simulink model "Project_model"  (R2024a)
settings: Solver=VariableStepAuto  StartTime=0.0  StopTime=Ts  RelTol=1e-4
values from neighbouring files (symbols this model uses):
  a = L/2    (= 1.385)    [IdeaI_vs_real_braking.m]    (also in Initialization_script.m)
  acc_pedal = 0    [Initialization_script.m]
  Af = 2.36    [Initialization_script.m]
  alpha = 0    [Initialization_script.m]
  b = L-a    (= 1.385)    [IdeaI_vs_real_braking.m]    (also in Initialization_script.m)
  brake_pedal = 1    [Initialization_script.m]
  Cx = 0.27    [Initialization_script.m]
  delay_acc = 0.02    [Initialization_script.m]
  delay_brake = 0.02    [Initialization_script.m]
  delay_release_acc = 30    [Initialization_script.m]
  delay_release_brake = 100    [Initialization_script.m]
  E_max = 58e3    (= 58000)    [Initialization_script.m]    (also in Power_losses.m)
  eff_engine = 0.90    (= 0.9)    [Caratteristica_coppia_rpm.m]    (also in Initialization_script.m)
  eff_transmission = 0.95    [Initialization_script.m]
  f0 = 0.009    [Initialization_script.m]
  f2 = 6.5e-6    (= 6.5e-06)    [Initialization_script.m]
  g = 9.81    [IdeaI_vs_real_braking.m]    (also in Initialization_script.m)
  gamma = 0    [Initialization_script.m]
  gear_ratio = 10.5    [Initialization_script.m]
  h = 0.55    [IdeaI_vs_real_braking.m]    (also in Initialization_script.m)
  Jns = 1    [Initialization_script.m]
  L = 2.77    [IdeaI_vs_real_braking.m]    (also in Initialization_script.m)
  lon_r = 0.055    [Initialization_script.m]    (also in Tyre215_50_19_Comb.m)
  m = 1812    [IdeaI_vs_real_braking.m]    (also in Initialization_script.m)
  max_braking_force = 15*m    (= 27180)    [Initialization_script.m]
  mu = 0.01:0.01:2    [IdeaI_vs_real_braking.m]    (also in Initialization_script.m = mmu(i))
  Pacn = Pace'    [Initialization_script.m]
  Radius = 0.35    [Initialization_script.m]    (also in Power_losses.m)
  regen_scaling = 1/10    (= 0.1)    [Initialization_script.m]
  rho = 1.29    [Initialization_script.m]
  SOC_init = 0.95    [Initialization_script.m]    (also in Power_losses.m)
  time_acc = 0    [Initialization_script.m]
  time_brake = 0    [Initialization_script.m]
  velstart = 100/3.6    (= 27.7777777778)    [Initialization_script.m]
libraries: cstblocks x2, simulink x1
settings Model: Creator=soffy  LastModifiedBy=luigi.maggipinto23
settings DataIOCC: ReturnWorkspaceOutputs=off
settings RTWCC: GPUComputeCapability=3.5

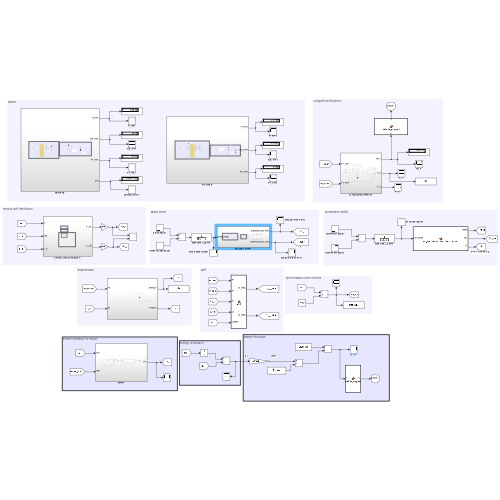
[thumbnail: Simulink's stored preview of the top-level diagram]
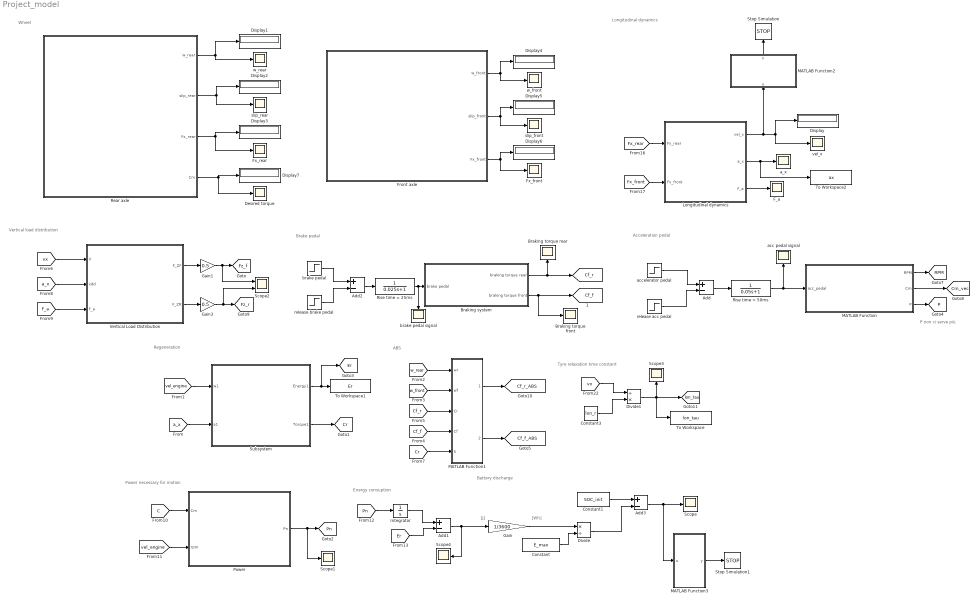
== system Project_model ==
  note: Battery discharge
  note: Energy consuption
  note: [J]
  note: [Wh]
  note: Power necessary for motion
  note: Tyre relaxation time constant
  note: Wheel
  note: Longitudinal dynamics
  note: P non ci serve più
  note: ABS
  note: Regeneration
  note: Acceleration pedal
  note: Vertical load distribution
  note: Brake pedal
  Add{,1..3} (4 alike) : Sum  Inputs=+-
  Braking system : Subsystem
  Braking torque front : Scope
  Braking torque rear : Scope
  Constant : Constant  Value=E_max
  Constant1 : Constant  Value=SOC_init
  Constant3 : Constant  Value=lon_r
  Desired torque : Scope
  Display{,1..7} (8 alike) : Display
  Divide : Product  Inputs=*/  RndMeth=Zero  SaturateOnIntegerOverflow=on
  Divide1 : Product  Inputs=/*
  F_a : Scope
  Front axle : Subsystem
  Fx_front : Scope
  Fx_rear : Scope
  Gain : Gain  Gain=1/3600
  Gain1 : Gain  Gain=0.5
  Gain3 : Gain  Gain=0.5
  Integrator : Integrator
  Longitudinal dynamics : Subsystem
  MATLAB Function : MATLAB Function  TreatAsAtomicUnit=on
  MATLAB Function1 : MATLAB Function  TreatAsAtomicUnit=on
  MATLAB Function2 : MATLAB Function  TreatAsAtomicUnit=on
  MATLAB Function3 : MATLAB Function  TreatAsAtomicUnit=on
  Power : Subsystem
  Rear axle : Subsystem
  Rise time = 25ms : TransferFcn  Denominator=[0.025 1]
  Rise time = 50ms : TransferFcn  Denominator=[0.05 1]
  Scope{,1,3..4} (4 alike) : Scope
  Scope2 : Scope  NumInputPorts=2
  Stop Simulation : Stop
  Stop Simulation1 : Stop
  Subsystem : Subsystem
  To Workspace : ToWorkspace  VariableName=lon_tau  SaveFormat=Timeseries  SampleTime=-1
  To Workspace1 : ToWorkspace  VariableName=Er  SaveFormat=Timeseries  SampleTime=-1
  To Workspace2 : ToWorkspace  VariableName=ax  SaveFormat=Timeseries  SampleTime=-1
  Vertical Load Distribution : Subsystem
  a_x : Scope
  acc pedal signal : Scope
  accelerator pedal : Step  Time=time_acc+delay_acc  After=acc_pedal  SampleTime=0
  brake pedal : Step  Time=time_brake+delay_brake  After=brake_pedal  SampleTime=0
  brake pedal signal : Scope
  release acc pedal : Step  Time=delay_release_acc+time_acc+delay_acc  After=acc_pedal  SampleTime=0
  release brake pedal : Step  Time=delay_release_brake+time_brake+delay_brake  After=brake_pedal  SampleTime=0
  slip_front : Scope
  slip_rear : Scope
  vel_x : Scope
  w_front : Scope
  w_rear : Scope
  tag scope: Cf_f=global, Cf_f_ABS=global, Cf_r=global, Cf_r_ABS=global, Cm_vec=global, Cr=global, Er=global, Fz_f=global, Fz_r=global, P=global, Pn=global, RPM=global, lon_tau=global
  wires:
  Braking system/1(braking torque rear) -> [Cf_r], Braking torque rear/1
  Vertical Load Distribution/1(F_ZF) -> Gain1/1
  Gain1/1 -> Scope2/1, [Fz_f]
  [vx] -> Vertical Load Distribution/1(V)
  [a_x] -> Vertical Load Distribution/2(xdd)
  [F_a] -> Vertical Load Distribution/3(F_a)
  Vertical Load Distribution/2(F_ZR) -> Gain3/1
  accelerator pedal/1 -> Add/1
  MATLAB Function/1(RPM) -> [RPM]
  MATLAB Function/2(Cm) -> [Cm_vec]
  Gain3/1 -> Scope2/2, [Fz_r]
  Braking system/2(braking torque front) -> Braking torque front/1, [Cf_f]
  Add/1 -> Rise time = 50ms/1
  [vel_engine] -> Subsystem/1(w1)
  [a_x] -> Subsystem/2(a1)
  MATLAB Function/3(P) -> [P]
  release acc pedal/1 -> Add/2
  Subsystem/1(Energy1) -> [Er], To Workspace1/1
  Subsystem/2(Torque1) -> [Cr]
  Rise time = 50ms/1 -> MATLAB Function/1(acc_pedal), acc pedal signal/1
  brake pedal/1 -> Add2/1
  release brake pedal/1 -> Add2/2
  Add2/1 -> Rise time = 25ms/1
  Rise time = 25ms/1 -> brake pedal signal/1, Braking system/1(brake pedal)
  [w_rear] -> MATLAB Function1/1(wr)
  [w_front] -> MATLAB Function1/2(wf)
  [Cf_r] -> MATLAB Function1/3(Cr)
  [Cf_f] -> MATLAB Function1/4(Cf)
  MATLAB Function1/1(Cr_ABS) -> [Cf_r_ABS]
  MATLAB Function1/2(Cf_ABS) -> [Cf_f_ABS]
  [Fx_rear] -> Longitudinal dynamics/1(Fx_rear)
  Longitudinal dynamics/2(a_x) -> To Workspace2/1, a_x/1
  Longitudinal dynamics/1(vel_x) -> MATLAB Function2/1(u), Display/1, vel_x/1
  [Fx_front] -> Longitudinal dynamics/2(Fx_front)
  Rear axle/1(w_rear) -> Display1/1, w_rear/1
  Rear axle/2(slip_rear) -> Display2/1, slip_rear/1
  Rear axle/3(Fx_rear) -> Display3/1, Fx_rear/1
  Front axle/1(w_front) -> Display4/1, w_front/1
  Front axle/2(slip_front) -> slip_front/1, Display5/1
  Front axle/3(Fx_front) -> Fx_front/1, Display6/1
  Longitudinal dynamics/3(F_a) -> F_a/1
  MATLAB Function2/1(y) -> Stop Simulation/1
  Rear axle/4(Cm) -> Desired torque/1, Display7/1
  [Cr] -> MATLAB Function1/5(Cregen)
  [vx] -> Divide1/1
  Constant3/1 -> Divide1/2
  Divide1/1 -> To Workspace/1, [lon_tau], Scope3/1
  [C] -> Power/1(Cm)
  [vel_engine] -> Power/2(rpm)
  [Pn] -> Integrator/1
  Integrator/1 -> Add1/1
  [Er] -> Add1/2
  Add1/1 -> Gain/1, Scope4/1
  Gain/1 -> Divide/1
  Constant/1 -> Divide/2
  Divide/1 -> Add3/2
  Constant1/1 -> Add3/1
  Add3/1 -> MATLAB Function3/1(u), Scope/1
  MATLAB Function3/1(y) -> Stop Simulation1/1
  Power/1(Pn) -> Scope1/1, [Pn]

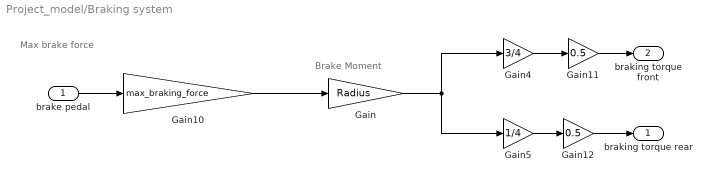
== system Project_model/Braking system ==
  note: Brake Moment
  note: Max brake force
  brake pedal : Inport
  Gain : Gain  Gain=Radius
  Gain10 : Gain  Gain=max_braking_force
  Gain11 : Gain  Gain=0.5
  Gain12 : Gain  Gain=0.5
  Gain4 : Gain  Gain=3/4
  Gain5 : Gain  Gain=1/4
  braking torque rear : Outport
  braking torque front : Outport  Port=2
  wires:
  brake pedal/1 -> Gain10/1
  Gain4/1 -> Gain11/1
  Gain5/1 -> Gain12/1
  Gain10/1 -> Gain/1
  Gain/1 -> Gain5/1, Gain4/1
  Gain12/1 -> braking torque rear/1
  Gain11/1 -> braking torque front/1

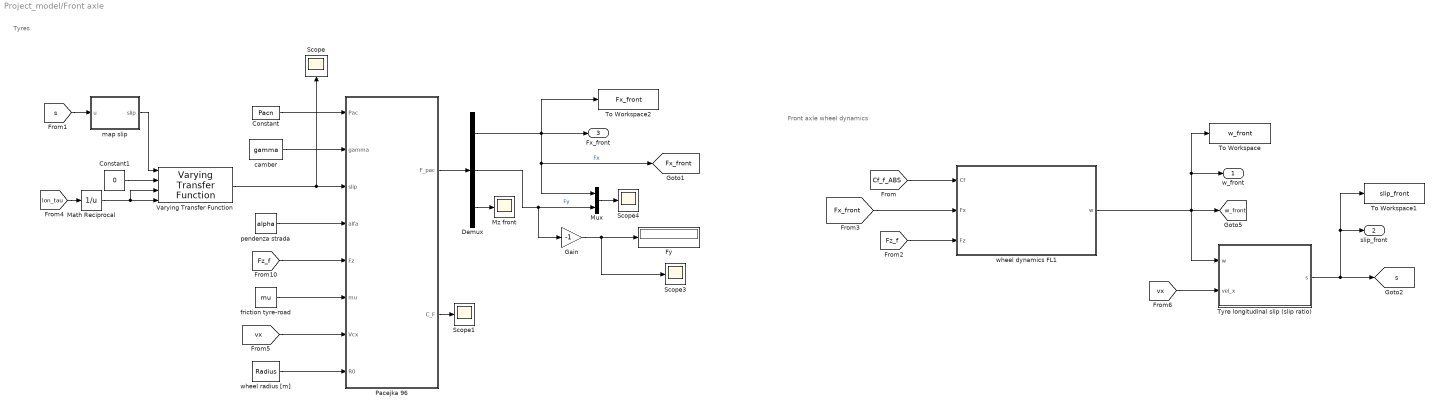
== system Project_model/Front axle ==
  note: Front axle wheel dynamics
  note: Tyres
  Constant : Constant  Value=Pacn
  Constant1 : Constant  Value=0
  Demux : Demux  Outputs=3
  Fy : Display
  Gain : Gain  Gain=-1
  Math Reciprocal : Math  Operator=reciprocal  SignedPower=on
  Mux : Mux  Inputs=2
  Mz front : Scope
  Pacejka 96 : MATLAB Function  TreatAsAtomicUnit=on
  Scope{,1,3..4} (4 alike) : Scope
  To Workspace : ToWorkspace  VariableName=w_front  SaveFormat=Timeseries  SampleTime=-1
  To Workspace1 : ToWorkspace  VariableName=slip_front  SaveFormat=Timeseries  SampleTime=-1
  To Workspace2 : ToWorkspace  VariableName=Fx_front  SaveFormat=Timeseries  SampleTime=-1
  Tyre longitudinal slip (slip ratio) : Subsystem
  Varying Transfer Function : cstblocks/Linear Parameter Varying/Varying Transfer Function  N=1  Feedthrough=on
  camber : Constant  Value=gamma
  friction tyre-road : Constant  Value=mu
  map slip : MATLAB Function  TreatAsAtomicUnit=on
  pendenza strada : Constant  Value=alpha
  wheel dynamics FL1 : Subsystem
  wheel radius [m] : Constant  Value=Radius
  w_front : Outport
  slip_front : Outport  Port=2
  Fx_front : Outport  Port=3
  tag scope: Fx_front=global, s=global, w_front=global
  wires:
  Mux/1 -> Scope4/1
  friction tyre-road/1 -> Pacejka 96/6(mu)
  [Fz_f] -> wheel dynamics FL1/3(Fz)
  Tyre longitudinal slip (slip ratio)/1(s) -> slip_front/1, To Workspace1/1, [s]
  Demux/1 -> To Workspace2/1, Fx_front/1, Mux/1, [Fx_front]  "Fx"
  Gain/1 -> Scope3/1, Fy/1
  Demux/3 -> Mz front/1
  wheel radius [m]/1 -> Pacejka 96/8(R0)
  wheel dynamics FL1/1(w) -> [w_front], w_front/1, To Workspace/1, Tyre longitudinal slip (slip ratio)/1(w)
  [vx] -> Pacejka 96/7(Vcx)
  Demux/2 -> Gain/1, Mux/2  "Fy"
  [Cf_f_ABS] -> wheel dynamics FL1/1(Cf)
  Constant/1 -> Pacejka 96/1(Pac)
  Pacejka 96/2(C_F) -> Scope1/1
  [s] -> map slip/1(u)
  camber/1 -> Pacejka 96/2(gamma)
  Pacejka 96/1(F_pac) -> Demux/1
  pendenza strada/1 -> Pacejka 96/4(alfa)
  [Fz_f] -> Pacejka 96/5(Fz)
  [Fx_front] -> wheel dynamics FL1/2(Fx)
  [vx] -> Tyre longitudinal slip (slip ratio)/2(vel_x)
  map slip/1(slip) -> Varying Transfer Function/1
  [lon_tau] -> Math Reciprocal/1
  Constant1/1 -> Varying Transfer Function/2
  Math Reciprocal/1 -> Varying Transfer Function/4, Varying Transfer Function/3
  Varying Transfer Function/1 -> Pacejka 96/3(slip), Scope/1

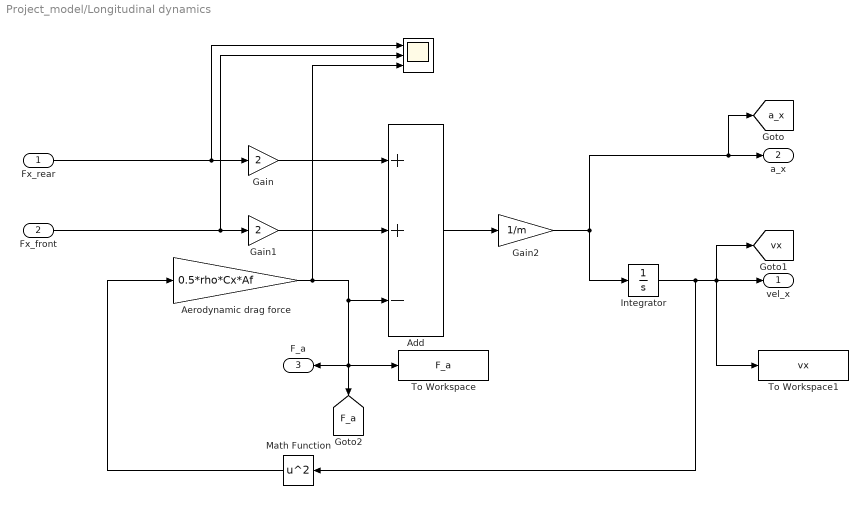
== system Project_model/Longitudinal dynamics ==
  Fx_rear : Inport
  Fx_front : Inport  Port=2
  " " : Scope  NumInputPorts=3
  Add : Sum  Inputs=++-
  Aerodynamic drag force : Gain  Gain=0.5*rho*Cx*Af
  Gain : Gain  Gain=2
  Gain1 : Gain  Gain=2
  Gain2 : Gain  Gain=1/m
  Integrator : Integrator  InitialCondition=velstart
  Math Function : Math  Operator=square  SignedPower=on  RndMeth=Zero
  To Workspace : ToWorkspace  VariableName=F_a  SaveFormat=Timeseries  SampleTime=-1
  To Workspace1 : ToWorkspace  VariableName=vx  SaveFormat=Timeseries  SampleTime=-1
  vel_x : Outport
  a_x : Outport  Port=2
  F_a : Outport  Port=3
  tag scope: F_a=global, a_x=global, vx=global
  wires:
  Integrator/1 -> To Workspace1/1, [vx], vel_x/1, Math Function/1
  Gain2/1 -> Integrator/1, [a_x], a_x/1
  Math Function/1 -> Aerodynamic drag force/1
  Gain/1 -> Add/1
  Add/1 -> Gain2/1
  Aerodynamic drag force/1 -> " "/3, Add/3, To Workspace/1, [F_a], F_a/1
  Fx_rear/1 -> Gain/1, " "/1
  Fx_front/1 -> " "/2, Gain1/1
  Gain1/1 -> Add/2

== system Project_model/Power ==
  note: potenza meccanica
  Cm : Inport
  rpm : Inport  Port=2
  Gain : Gain  Gain=2*pi/60
  MATLAB Function3 : MATLAB Function  TreatAsAtomicUnit=on
  Product : Product
  Pn : Outport
  wires:
  Gain/1 -> Product/2
  rpm/1 -> Gain/1
  Cm/1 -> Product/1
  Product/1 -> MATLAB Function3/1(P_mechanic)
  MATLAB Function3/1(P_electric) -> Pn/1

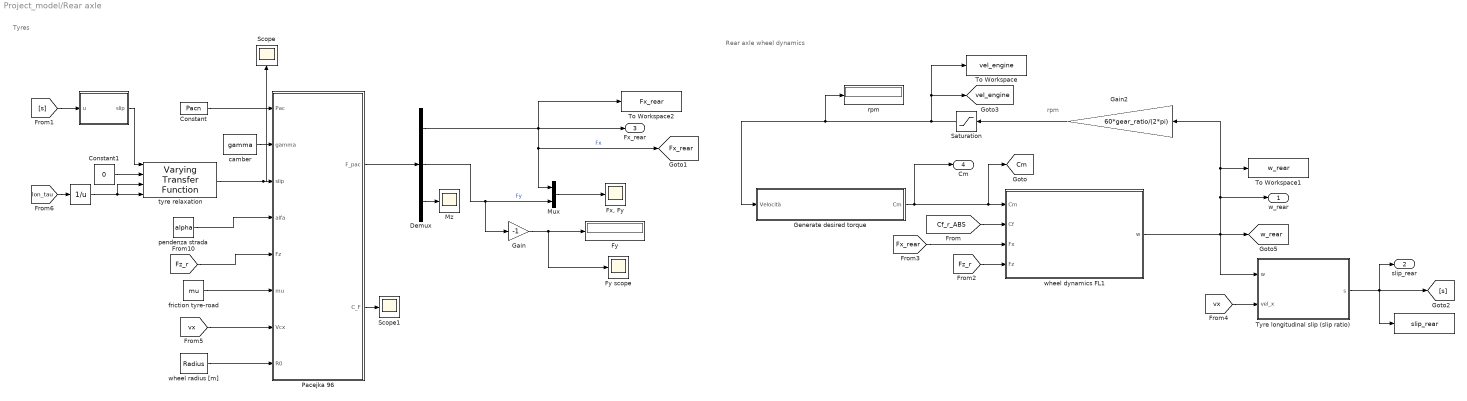
== system Project_model/Rear axle ==
  note: Rear axle wheel dynamics
  note: Tyres
  note: rpm
  " " : ToWorkspace  VariableName=slip_rear  SaveFormat=Timeseries  SampleTime=-1
  "  " : MATLAB Function  TreatAsAtomicUnit=on
  "    " : Math  Operator=reciprocal  SignedPower=on
  Constant : Constant  Value=Pacn
  Constant1 : Constant  Value=0
  Demux : Demux  Outputs=3
  "Fx, Fy" : Scope
  Fy : Display
  Fy scope : Scope
  Gain : Gain  Gain=-1
  Gain2 : Gain  Gain=60*gear_ratio/(2*pi)
  Generate desired torque : Subsystem
  Mux : Mux  Inputs=2
  Mz : Scope
  Pacejka 96 : MATLAB Function  TreatAsAtomicUnit=on
  Saturation : Saturate  UpperLimit=16000  LowerLimit=-16000
  Scope : Scope
  Scope1 : Scope
  To Workspace : ToWorkspace  VariableName=vel_engine  SaveFormat=Timeseries  SampleTime=-1
  To Workspace1 : ToWorkspace  VariableName=w_rear  SaveFormat=Timeseries  SampleTime=-1
  To Workspace2 : ToWorkspace  VariableName=Fx_rear  SaveFormat=Timeseries  SampleTime=-1
  Tyre longitudinal slip (slip ratio) : Subsystem
  camber : Constant  Value=gamma
  friction tyre-road : Constant  Value=mu
  pendenza strada : Constant  Value=alpha
  rpm : Display
  tyre relaxation : cstblocks/Linear Parameter Varying/Varying Transfer Function  N=1  Feedthrough=on
  wheel dynamics FL1 : Subsystem
  wheel radius [m] : Constant  Value=Radius
  w_rear : Outport
  slip_rear : Outport  Port=2
  Fx_rear : Outport  Port=3
  Cm : Outport  Port=4
  tag scope: Cm=global, Fx_rear=global, vel_engine=global, w_rear=global
  wires:
  Mux/1 -> "Fx, Fy"/1
  friction tyre-road/1 -> Pacejka 96/6(mu)
  [Fz_r] -> wheel dynamics FL1/4(Fz)
  Tyre longitudinal slip (slip ratio)/1(s) -> " "/1, slip_rear/1, [s]
  Gain/1 -> Fy/1, Fy scope/1
  Demux/3 -> Mz/1
  Generate desired torque/1(Cm) -> Cm/1, [Cm], wheel dynamics FL1/1(Cm)
  wheel radius [m]/1 -> Pacejka 96/8(R0)
  Saturation/1 -> [vel_engine], To Workspace/1, rpm/1, Generate desired torque/1(Velocità)
  wheel dynamics FL1/1(w) -> To Workspace1/1, Gain2/1, w_rear/1, [w_rear], Tyre longitudinal slip (slip ratio)/1(w)
  [vx] -> Pacejka 96/7(Vcx)
  Demux/2 -> Gain/1, Mux/2  "Fy"
  Constant/1 -> Pacejka 96/1(Pac)
  Gain2/1 -> Saturation/1
  Pacejka 96/2(C_F) -> Scope1/1
  [s] -> "  "/1(u)
  camber/1 -> Pacejka 96/2(gamma)
  Pacejka 96/1(F_pac) -> Demux/1
  pendenza strada/1 -> Pacejka 96/4(alfa)
  [Fz_r] -> Pacejka 96/5(Fz)
  [Fx_rear] -> wheel dynamics FL1/3(Fx)
  [Cf_r_ABS] -> wheel dynamics FL1/2(Cf)
  [vx] -> Tyre longitudinal slip (slip ratio)/2(vel_x)
  Constant1/1 -> tyre relaxation/2
  "    "/1 -> tyre relaxation/3, tyre relaxation/4
  [lon_tau] -> "    "/1
  tyre relaxation/1 -> Scope/1, Pacejka 96/3(slip)
  Demux/1 -> To Workspace2/1, Fx_rear/1, Mux/1, [Fx_rear]  "Fx"
  "  "/1(slip) -> tyre relaxation/1

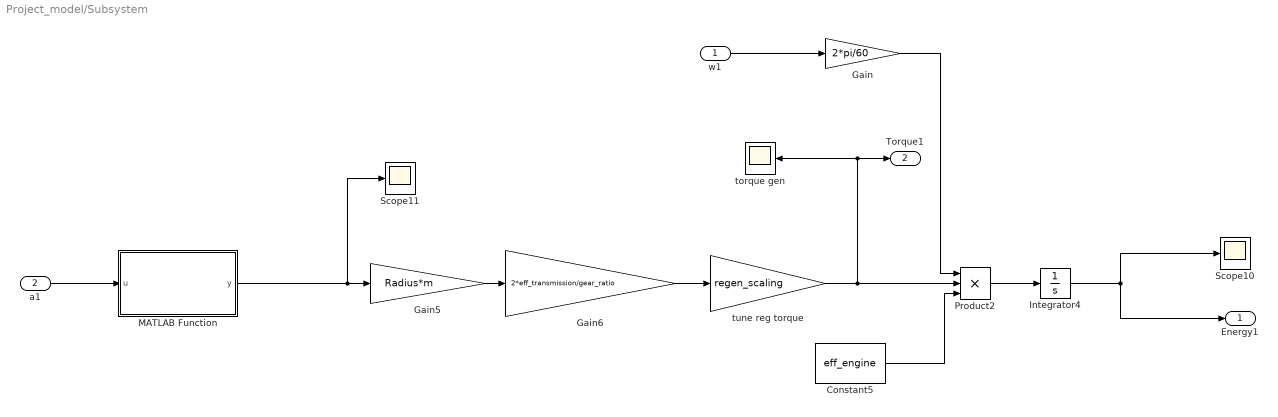
== system Project_model/Subsystem ==
  w1 : Inport
  a1 : Inport  Port=2
  Constant5 : Constant  Value=eff_engine
  Gain : Gain  Gain=2*pi/60
  Gain5 : Gain  Gain=Radius*m
  Gain6 : Gain  Gain=2*eff_transmission/gear_ratio
  Integrator4 : Integrator
  MATLAB Function : MATLAB Function  TreatAsAtomicUnit=on
  Product2 : Product  Inputs=3
  Scope10 : Scope
  Scope11 : Scope
  torque gen : Scope
  tune reg torque : Gain  Gain=regen_scaling
  Energy1 : Outport
  Torque1 : Outport  Port=2
  wires:
  Product2/1 -> Integrator4/1
  Constant5/1 -> Product2/3
  w1/1 -> Gain/1
  Integrator4/1 -> Scope10/1, Energy1/1
  Gain5/1 -> Gain6/1
  a1/1 -> MATLAB Function/1(u)
  MATLAB Function/1(y) -> Scope11/1, Gain5/1
  Gain6/1 -> tune reg torque/1
  tune reg torque/1 -> Torque1/1, torque gen/1, Product2/2
  Gain/1 -> Product2/1

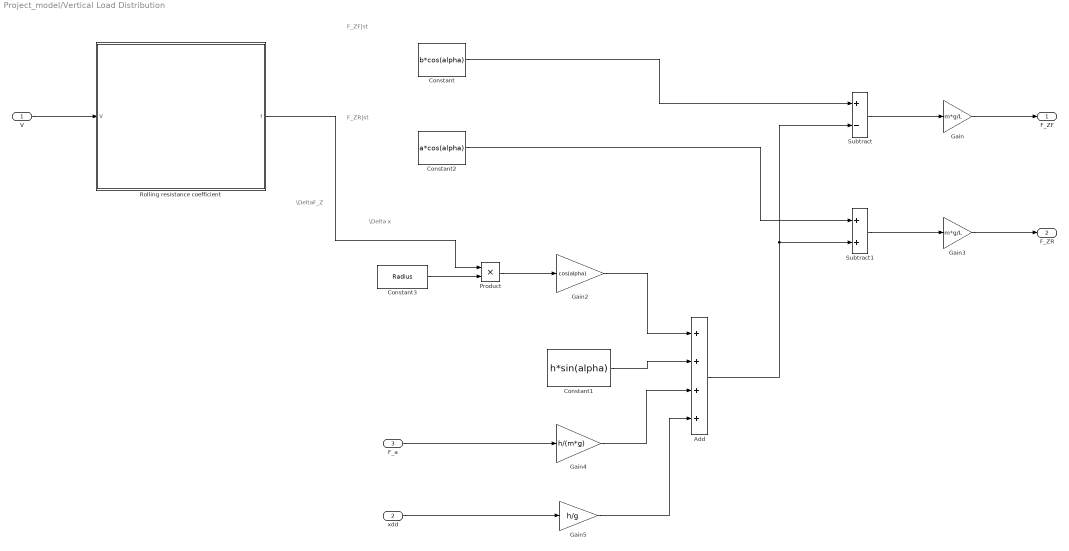
== system Project_model/Vertical Load Distribution ==
  note: \Delta x
  note: \DeltaF_Z
  note: F_ZR|st
  note: F_ZF|st
  V : Inport
  xdd : Inport  Port=2
  F_a : Inport  Port=3
  Add : Sum  Inputs=++++
  Constant : Constant  Value=b*cos(alpha)
  Constant1 : Constant  Value=h*sin(alpha)
  Constant2 : Constant  Value=a*cos(alpha)
  Constant3 : Constant  Value=Radius
  Gain : Gain  Gain=m*g/L
  Gain2 : Gain  Gain=cos(alpha)
  Gain3 : Gain  Gain=m*g/L
  Gain4 : Gain  Gain=h/(m*g)
  Gain5 : Gain  Gain=h/g
  Product : Product
  Rolling resistance coefficient : Subsystem
  Subtract : Sum  Inputs=+-
  Subtract1 : Sum
  F_ZF : Outport
  F_ZR : Outport  Port=2
  wires:
  Subtract1/1 -> Gain3/1
  xdd/1 -> Gain5/1
  Gain3/1 -> F_ZR/1
  Constant1/1 -> Add/2
  Add/1 -> Subtract1/2, Subtract/2
  Gain/1 -> F_ZF/1
  V/1 -> Rolling resistance coefficient/1(V)
  Gain5/1 -> Add/4
  Gain4/1 -> Add/3
  Gain2/1 -> Add/1
  Constant/1 -> Subtract/1
  Subtract/1 -> Gain/1
  F_a/1 -> Gain4/1
  Constant2/1 -> Subtract1/1
  Product/1 -> Gain2/1
  Rolling resistance coefficient/1(f) -> Product/1
  Constant3/1 -> Product/2

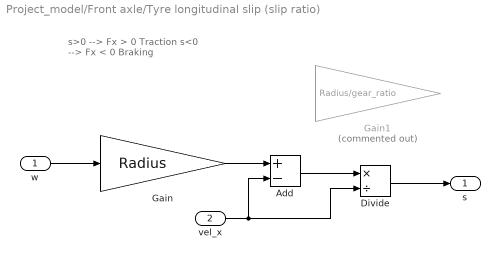
== system Project_model/Front axle/Tyre longitudinal slip (slip ratio) ==
  note: s>0 --> Fx > 0 Traction
      | s<0 --> Fx < 0 Braking
  w : Inport
  vel_x : Inport  Port=2
  Add : Sum  Inputs=+-
  Divide : Product  Inputs=*/
  Gain : Gain  Gain=Radius
  Gain1 : Gain  Commented=on  Gain=Radius/gear_ratio
  s : Outport
  wires:
  vel_x/1 -> Divide/2, Add/2
  Add/1 -> Divide/1
  Divide/1 -> s/1
  Gain/1 -> Add/1
  w/1 -> Gain/1

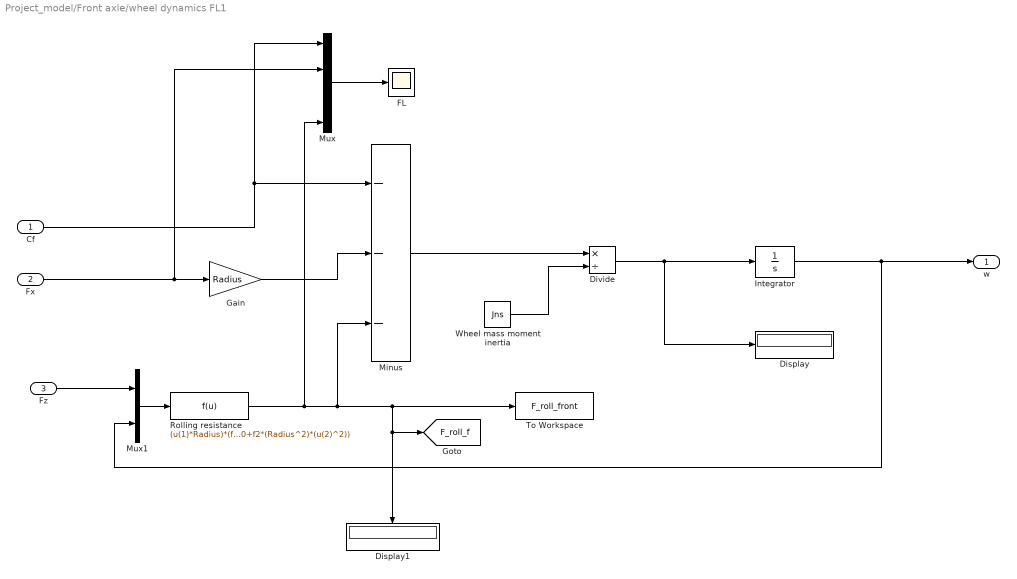
== system Project_model/Front axle/wheel dynamics FL1 ==
  Cf : Inport
  Fx : Inport  Port=2
  Fz : Inport  Port=3
  Display : Display
  Display1 : Display
  Divide : Product  Inputs=*/
  FL : Scope
  Gain : Gain  Gain=Radius
  Integrator : Integrator  InitialCondition=velstart/Radius
  Minus : Sum  Inputs=---
  Mux : Mux
  Mux1 : Mux  Inputs=2
  Rolling resistance : Fcn  Expr=(u(1)*Radius)*(f0+f2*(Radius^2)*(u(2)^2))
  To Workspace : ToWorkspace  VariableName=F_roll_front  SaveFormat=Timeseries  SampleTime=-1
  Wheel mass moment inertia : Constant  Value=Jns
  w : Outport
  tag scope: F_roll_f=global
  wires:
  Cf/1 -> Mux/1, Minus/1
  Fx/1 -> Mux/2, Gain/1
  Mux/1 -> FL/1
  Fz/1 -> Mux1/1
  Minus/1 -> Divide/1
  Integrator/1 -> w/1, Mux1/2
  Wheel mass moment inertia/1 -> Divide/2
  Mux1/1 -> Rolling resistance/1
  Gain/1 -> Minus/2
  Rolling resistance/1 -> Minus/3, Display1/1, [F_roll_f], To Workspace/1, Mux/4
  Divide/1 -> Integrator/1, Display/1

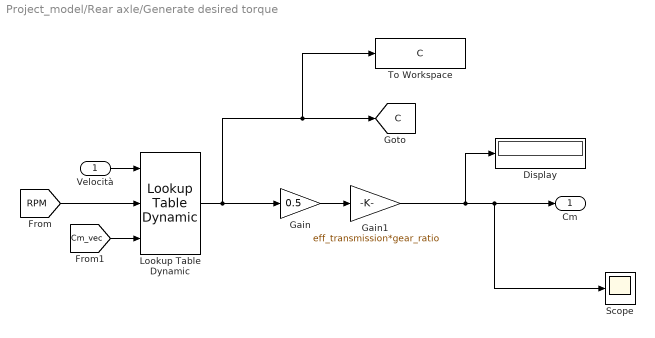
== system Project_model/Rear axle/Generate desired torque ==
  Velocità : Inport
  Display : Display
  Gain : Gain  Gain=0.5
  Gain1 : Gain  Gain=eff_transmission*gear_ratio
  Lookup Table Dynamic : simulink/Lookup Tables/Lookup Table Dynamic  LookUpMeth=Interpolation-Use End Values  OutDataType=fixdt('double')  OutScaling=[]  OutputDataTypeScalingMode=Specify via dialog  OutDataTypeStr=double  DoSatur=off
  Scope : Scope
  To Workspace : ToWorkspace  VariableName=C  SaveFormat=Timeseries  SampleTime=-1
  Cm : Outport
  tag scope: C=global
  wires:
  Velocità/1 -> Lookup Table Dynamic/1
  Lookup Table Dynamic/1 -> To Workspace/1, [C], Gain/1
  Gain/1 -> Gain1/1
  [Cm_vec] -> Lookup Table Dynamic/3
  [RPM] -> Lookup Table Dynamic/2
  Gain1/1 -> Display/1, Scope/1, Cm/1

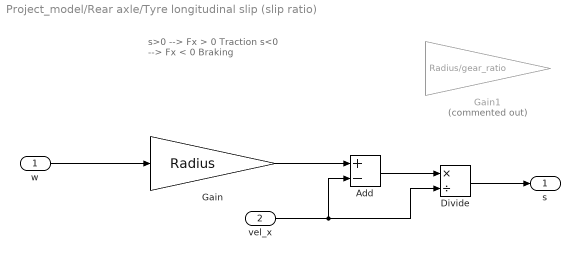
== system Project_model/Rear axle/Tyre longitudinal slip (slip ratio) ==
  note: s>0 --> Fx > 0 Traction
      | s<0 --> Fx < 0 Braking
  w : Inport
  vel_x : Inport  Port=2
  Add : Sum  Inputs=+-
  Divide : Product  Inputs=*/
  Gain : Gain  Gain=Radius
  Gain1 : Gain  Commented=on  Gain=Radius/gear_ratio
  s : Outport
  wires:
  vel_x/1 -> Divide/2, Add/2
  Add/1 -> Divide/1
  Divide/1 -> s/1
  w/1 -> Gain/1
  Gain/1 -> Add/1

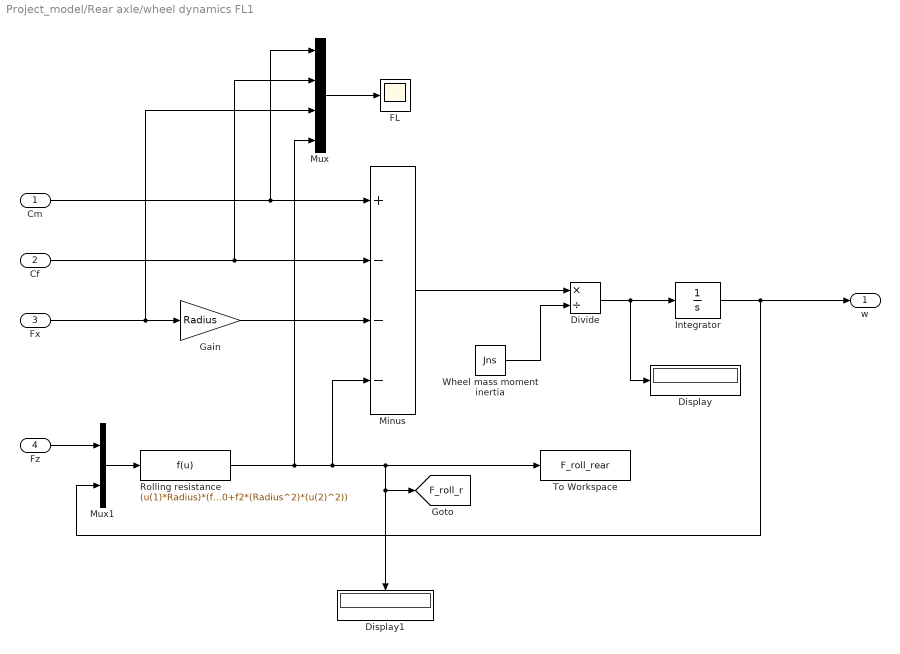
== system Project_model/Rear axle/wheel dynamics FL1 ==
  Cm : Inport
  Cf : Inport  Port=2
  Fx : Inport  Port=3
  Fz : Inport  Port=4
  Display : Display
  Display1 : Display
  Divide : Product  Inputs=*/
  FL : Scope
  Gain : Gain  Gain=Radius
  Integrator : Integrator  InitialCondition=velstart/Radius
  Minus : Sum  Inputs=+---
  Mux : Mux
  Mux1 : Mux  Inputs=2
  Rolling resistance : Fcn  Expr=(u(1)*Radius)*(f0+f2*(Radius^2)*(u(2)^2))
  To Workspace : ToWorkspace  VariableName=F_roll_rear  SaveFormat=Timeseries  SampleTime=-1
  Wheel mass moment inertia : Constant  Value=Jns
  w : Outport
  tag scope: F_roll_r=global
  wires:
  Cm/1 -> Mux/1, Minus/1
  Fx/1 -> Gain/1, Mux/3
  Mux/1 -> FL/1
  Fz/1 -> Mux1/1
  Rolling resistance/1 -> Mux/4, [F_roll_r], Display1/1, To Workspace/1, Minus/4
  Divide/1 -> Display/1, Integrator/1
  Minus/1 -> Divide/1
  Integrator/1 -> w/1, Mux1/2
  Wheel mass moment inertia/1 -> Divide/2
  Mux1/1 -> Rolling resistance/1
  Gain/1 -> Minus/3
  Cf/1 -> Mux/2, Minus/2

== system Project_model/Vertical Load Distribution/Rolling resistance coefficient ==
  V : Inport
  Add : Sum
  Constant3 : Constant  Value=f0
  Constant4 : Constant  Value=f2
  Product : Product
  Square : Math  Operator=square
  f : Outport
  wires:
  V/1 -> Square/1
  Constant3/1 -> Add/1
  Constant4/1 -> Product/2
  Square/1 -> Product/1
  Product/1 -> Add/2
  Add/1 -> f/1

== matlab function Project_model/MATLAB Function3 ==
  data: u input; y output
function y = vehicle_stopped(u)

y = 0;
if u <= 0
    y = 1;
end

== matlab function Project_model/Rear axle/Pacejka 96 ==
  settings: fimath=|
      | fimath(...
      | 'RoundMode', 'floor',...
      | 'OverflowMode', 'wrap',...
      | 'ProductMode', 'KeepLSB', 'ProductWordLength', 32,...
      | 'SumMode', 'KeepLSB', 'SumWordLength', 32,...
      | 'CastBeforeSum', false)
  data: Pac input; gamma input; slip input; alfa input; Fz input; F_pac output; mu input; Vcx input; C_F output; R0 input
function [F_pac,C_F] = fcn(Pac,gamma,slip,alfa,Fz,mu,Vcx,R0)
% function for computing forces Fx, Fy and self-aligning torque Mz

% Pac   -> model structure with coeff. Pacejka 96
% slip  -> slip ratio [-] (-1:1)
% alfa  -> slip angle [rad]
% gamma -> camber [rad]
% Vcx,y velocity components of tire contact point C

% Structure building: Pacejka model coefficients
Pa_FZ0_ = Pac(1);
Pa_LFZ0 = Pac(2);
Pa_LmuV = Pac(3);
Pa_LKXK = Pac(4);
Pa_LKYA = Pac(5);
Pa_LCX_ = Pac(6);
Pa_LCY_ = Pac(7);
Pa_LEX_ = Pac(8);
Pa_LEY_ = Pac(9);
Pa_LHX_ = Pac(10);
Pa_LHY_ = Pac(11);
Pa_LVX_ = Pac(12);
Pa_LVY_ = Pac(13);
Pa_LKYG = Pac(14);
Pa_LKZG = Pac(15);
Pa_LT__ = Pac(16);
Pa_MR__ = Pac(17);
Pa_LXA_ = Pac(18);
Pa_LYK_ = Pac(19);
Pa_LVYK = Pac(20);
Pa_LS__ = Pac(21);
Pa_LCZ_ = Pac(22);
Pa_LMX_ = Pac(23);
Pa_LMY_ = Pac(24);
Pa_PCX1 = Pac(25);
Pa_PDX1 = Pac(26);
Pa_PDX2 = Pac(27);
Pa_PEX1 = Pac(28);
Pa_PEX2 = Pac(29);
Pa_PEX3 = Pac(30);
Pa_PEX4 = Pac(31);
Pa_PKX1 = Pac(32);
Pa_PKX2 = Pac(33);
Pa_PKX3 = Pac(34);
Pa_PHX1 = Pac(35);
Pa_PHX2 = Pac(36);
Pa_PVX1 = Pac(37);
Pa_PVX2 = Pac(38);
Pa_RBX1 = Pac(39);
Pa_RBX2 = Pac(40);
Pa_RCX1 = Pac(41);
Pa_RHX1 = Pac(42);
Pa_RTX1 = Pac(43);
Pa_RTX2 = Pac(44);
Pa_RTX3 = Pac(45);
Pa_QSX1 = Pac(46);
Pa_QSX2 = Pac(47);
Pa_QSX3 = Pac(48);
Pa_PCY1 = Pac(49);
Pa_PDY1 = Pac(50);
Pa_PDY2 = Pac(51);
Pa_PDY3 = Pac(52);
Pa_PEY1 = Pac(53);
Pa_PEY2 = Pac(54);
Pa_PEY3 = Pac(55);
Pa_PEY4 = Pac(56);
Pa_PKY1 = Pac(57);
Pa_PKY2 = Pac(58);
Pa_PKY3 = Pac(59);
Pa_PHY1 = Pac(60);
Pa_PHY2 = Pac(61);
Pa_PHY3 = Pac(62);
Pa_PVY1 = Pac(63);
Pa_PVY2 = Pac(64);
Pa_PVY3 = Pac(65);
Pa_PVY4 = Pac(66);
Pa_RBY1 = Pac(67);
Pa_RBY2 = Pac(68);
Pa_RBY3 = Pac(69);
Pa_RCY1 = Pac(70);
Pa_RHY1 = Pac(71);
Pa_RVY1 = Pac(72);
Pa_RVY2 = Pac(73);
Pa_RVY3 = Pac(74);
Pa_RVY4 = Pac(75);
Pa_RVY5 = Pac(76);
Pa_RVY6 = Pac(77);
Pa_PTY1 = Pac(78);
Pa_PTY2 = Pac(79);
Pa_QSY1 = Pac(80);
Pa_QSY2 = Pac(81);
Pa_QBZ1 = Pac(82);
Pa_QBZ2 = Pac(83);
Pa_QBZ3 = Pac(84);
Pa_QBZ4 = Pac(85);
Pa_QBZ5 = Pac(86);
Pa_QBZ6 = Pac(87);
Pa_QBZ9 = Pac(88);
Pa_QBZZ = Pac(89);
Pa_QCZ1 = Pac(90);
Pa_QDZ1 = Pac(91);
Pa_QDZ2 = Pac(92);
Pa_QDZ3 = Pac(93);
Pa_QDZ4 = Pac(94);
Pa_QDZ6 = Pac(95);
Pa_QDZ7 = Pac(96);
Pa_QDZ8 = Pac(97);
Pa_QDZ9 = Pac(98);
Pa_QEZ1 = Pac(99);
Pa_QEZ2 = Pac(100);
Pa_QEZ3 = Pac(101);
Pa_QEZ4 = Pac(102);
Pa_QEZ5 = Pac(103);
Pa_QHZ1 = Pac(104);
Pa_QHZ2 = Pac(105);
Pa_QHZ3 = Pac(106);
Pa_QHZ4 = Pac(107);
Pa_SSZ1 = Pac(108);
Pa_SSZ2 = Pac(109);
Pa_SSZ3 = Pac(110);
Pa_SSZ4 = Pac(111);
Pa_QTZ1 = Pac(112);

% Costants
epsi = 0.01;
eps_V = 0.1;
csi_0=1;
csi_4=1;
Amu = 10;
Pa_LmuX = mu;
Pa_LmuY = mu;

%-------------------------------- Fx pure slip ---------------------------
Cx = Pa_PCX1*Pa_LCX_;
dfz = (Fz-Pa_LFZ0*Pa_FZ0_)/(Pa_LFZ0*Pa_FZ0_);
mux = Pa_LmuX * (Pa_PDX1 + Pa_PDX2 * dfz);
Dx = mux*Fz; %*csi_1, con csi_1=1
%Shx = (Pa_PHX1+Pa_PHX2*dfz)*Pa_LHX_;
Shx = 0;
Kx = slip + Shx;
Ex = (Pa_PEX1+Pa_PEX2*dfz+Pa_PEX3*dfz^2)*(1-Pa_PEX4*sign(Kx))*Pa_LEX_;
if Ex>1 Et=1; end
Kxk = Fz*(Pa_PKX1+Pa_PKX2*dfz)*exp(Pa_PKX3*dfz)*Pa_LKXK;
Bx = Kxk/(Cx*Dx+epsi);
lam_mux  = Pa_LmuX*Amu/(1+(Amu-1)*Pa_LmuX);
SVx = Fz*(Pa_PVX1+Pa_PVX2*dfz)*(abs(Vcx)/(abs(Vcx)+eps_V))*Pa_LVX_*lam_mux; %*csi_1, con csi_1=1

% logitudinal slip stiffness (Fx slope in the origin)
C_Fk = Bx*Cx*Dx;

% longitudinal force
Fx0 = Dx*sin(Cx*atan(Bx*Kx-Ex*(Bx*Kx-atan(Bx*Kx)))) + SVx;

%---------------------------- Fy pure side slip --------------------------
seg=sign(Vcx);
if seg==0 seg=1; end
alfa_star = tan(alfa)*seg;
gam_star = sin(gamma);
Shy = (Pa_PHY1+Pa_PHY2*dfz)*Pa_LHY_+Pa_PHY3*gam_star*Pa_LKYG*csi_0+csi_4-1;
alfa_y = alfa_star + Shy;
Cy = Pa_PCY1*Pa_LCY_;
muy = Pa_LmuY*(Pa_PDY1+Pa_PDY2*dfz)*(1-Pa_PDY3*gam_star^2);
Dy = muy*Fz; %*csi_2, con csi_2=1
Ey = (Pa_PEY1+Pa_PEY2*dfz)*(1-(Pa_PEY3+Pa_PEY4*gam_star)*sign(alfa_y))*Pa_LEY_;
if Ey>1 Ey=1; end
Kya0 = Pa_PKY1*Pa_LFZ0*Pa_FZ0_*sin(2*atan(Fz/(Pa_PKY2*Pa_LFZ0*Pa_FZ0_)))*Pa_LKYA;
Kya = Kya0*(1-Pa_PKY3*gam_star^2); %*csi_3, con csi_3=1
By = Kya/(Cy*Dy+epsi);
lam_muy = Pa_LmuY*Amu/(1+(Amu-1)*Pa_LmuY);
SVy = Fz*((Pa_PVY1+Pa_PVY2*dfz)*Pa_LVY_+(Pa_PVY3+Pa_PVY4*dfz)*gam_star*Pa_LKYG )*lam_muy; %*csi_2, con csi_2=1
Kyg0 = (Pa_PHY3*Kya0+Fz*(Pa_PVY3+Pa_PVY4*dfz))*Pa_LKYG;

% cornering stiffness (Fy slope in the origin)
C_Fa = By*Cy*Dy;

% lateral force
Fy0 = Dy*sin(Cy*atan(By*alfa_y-Ey*(By*alfa_y-atan(By*alfa_y)))) + SVy;

% --------------------- Fx combined slip ------------------------------
Shxa = Pa_RHX1;
%Exa = Pa_REX1+Pa_REX2*dfz; NON esiste Pa.REX1 ne' Pa.REX2
Exa = 0;
Cxa = Pa_RCX1;
Bxa = Pa_RBX1*cos(atan(Pa_RBX2*slip))*Pa_LXA_;
alfaS = alfa_star+Shxa;
Gxa0 = cos(Cxa*atan(Bxa*Shxa-Exa*(Bxa*Shxa-atan(Bxa*Shxa))));
Gxa = cos(Cxa*atan(Bxa*alfaS-Exa*(Bxa*alfaS-atan(Bxa*alfaS))))/Gxa0;
Fx = Fx0*Gxa;

% ---------------------- Fy combined slip ------------------------------
Dvyk = muy*Fz*(Pa_RVY1+Pa_RVY2*dfz+Pa_RVY3*gam_star)*cos(atan(Pa_RVY4*alfa_star));%*csi_2, con csi_2=1
Svyk = Dvyk*sin(Pa_RVY5*atan(Pa_RVY6*slip));
Shyk = Pa_RHY1; %+Pa.RHY2*dfz; NON esiste Pa.RHY2
Cyk = Pa_RCY1;
Byk = Pa_RBY1*cos(atan(Pa_RBY2*(alfa_star-Pa_RBY3)))*Pa_LYK_;
%Eyk = Pa_REY1+Pa_REY2*dfz; NON esiste Pa.REY1 ne' Pa.REY2
Eyk = 0;
ks = slip+Shyk;
Gyk0 = cos(Cyk*atan(Byk*Shyk-Eyk*(Byk*Shyk-atan(Byk*Shyk))));
Gyk = cos(Cyk*atan(Byk*ks-Eyk*(Byk*ks-atan(Byk*ks))))/Gyk0;
Fy = Fy0*Gyk+Svyk;

% --------------------- Mz pure side slip  ---------------------------
Shf = Shy+SVy/Kya;
alfa_r = alfa_star+Shf;
Br = (Pa_QBZ9/Pa_LmuY+Pa_QBZZ*By*Cy); %*csi_6, con csi_6=1
%%% Pa_QBZZ e' in realta' QBZ10 scritto cosi' x ragioni di spazio
Cr = 1; %*csi_7, con csi_7=1
Dr = Fz*R0*((Pa_QDZ6+Pa_QDZ7*dfz)+(Pa_QDZ8+Pa_QDZ9*dfz)*gam_star)*cos(alfa)*Pa_LmuY*seg; %+csi_8-1, con csi_8=1
Mzr0 = Dr*cos(Cr*atan(Br*alfa_r));
Sht = Pa_QHZ1+Pa_QHZ2*dfz+(Pa_QHZ3+Pa_QHZ4*dfz)*gam_star;
alfa_t = alfa_star+Sht;
Bt = (Pa_QBZ1+Pa_QBZ2*dfz+Pa_QBZ3*dfz^2)*(1+Pa_QBZ5*abs(gam_star)+Pa_QBZ6*gam_star^2)*Pa_LKYA/Pa_LmuY;
if Bt<0 Bt=0; end
Ct = Pa_QCZ1;
Dt0 = Fz*R0/(Pa_LFZ0*Pa_FZ0_)*(Pa_QDZ1+Pa_QDZ2*dfz)*seg;
Dt = Dt0*(1+Pa_QDZ3*abs(gam_star)+Pa_QDZ4*gam_star^2); %*csi_5, con csi_5=1
Et = (Pa_QEZ1+Pa_QEZ2*dfz+Pa_QEZ3*dfz^2)*(1+(Pa_QEZ4+Pa_QEZ5*gam_star)*2/pi*atan(Bt*Ct*alfa_t));
if Et>1 Et=1; end
t0 = Dt*cos(Ct*atan(Bt*alfa_t - Et*(Bt*alfa_t-atan(Bt*alfa_t))))*cos(alfa);
Mz0 = -t0*Fy;
Kza0 = Dt0*Kya0;
%Kzg0 = Fz*R0*(Pa_QDZ8+Pa_QDZ9*dfz)-Dt0*Kyg0;

% aligning torque
Mz = Mz0 + Mzr0;

% ------------------------ Mz Combined -----------------------------
eps_k = 0; % 
lambda_s = Pa_LS__ ;
Fz0p = Pa_LFZ0*Pa_FZ0_;
K_yap = Kya + eps_k;
alfa_req = sqrt(alfa_r^2+(Kxk/K_yap)^2*slip^2)*sign(alfa_r);
alfa_teq = sqrt(alfa_t^2+(Kxk/K_yap)^2*slip^2)*sign(alfa_t);
s = R0*(Pa_SSZ1 + Pa_SSZ2*(Fy/Fz0p) + (Pa_SSZ3+Pa_SSZ4*dfz)*gam_star)*lambda_s;
Mzr = Dr*cos(Cr*atan(Br*alfa_req));
Fyp = Fy-Svyk; 
t = Dt*cos(Ct*atan(Bt*alfa_teq - Et*(Bt*alfa_teq-atan(Bt*alfa_teq))))*cos(alfa);
Mzp = -t*Fyp;
% aligning torque
Mz = Mzp + Mzr + s*Fx;
%%%%%%%%%%%%%%%%%%%%%%%

% Check that Fz is positive
if Fz <= 0
    Fx = 0;
    Fy = 0;
    Mz = 0;
end

% Output
F_pac = [Fx; Fy; Mz];
C_F = [C_Fk; C_Fa];

== matlab function Project_model/Rear axle/   ==
  data: u input; slip output
function slip = adjust_slip(u)

if isnan(u) || isinf(u)
    slip = 0;
else
    slip = u;
end

== matlab function Project_model/MATLAB Function ==
  data: acc_pedal input; RPM output; Cm output; P output
function [RPM, Cm, P]  = engine_vel_torque_characteristic(acc_pedal)

% Parameters
P_max = 150e3; % [W]
C_max = 310; % [Nm]
RPM_max = 16000; % max speed [rpm]
P_batt = P_max * acc_pedal;

% Efficiency 
eff_engine = 0.90;

P_motore = P_batt * eff_engine;
C_motore= (acc_pedal * C_max) * eff_engine; 

% Parametri del motore elettrico
RPM_bar = P_motore * 60 / (2 * pi * C_motore); % RPM corrispondenti a P_max e C_max

% RPM da 0 a 16000
RPM = linspace(0, RPM_max, 1000);

% Calcolo di C
C = zeros(size(RPM));
C(RPM <= RPM_bar) = C_motore;
C(RPM > RPM_bar) = (P_motore * 60) ./ (2 * pi * RPM(RPM > RPM_bar));

Cm = C;

% Calcolo di P
P = zeros(size(RPM));
P(RPM <= RPM_bar) = (P_motore / RPM_bar) * RPM(RPM <= RPM_bar);
P(RPM > RPM_bar) = P_motore;

== matlab function Project_model/Front axle/Pacejka 96 ==
  settings: fimath=|
      | fimath(...
      | 'RoundMode', 'floor',...
      | 'OverflowMode', 'wrap',...
      | 'ProductMode', 'KeepLSB', 'ProductWordLength', 32,...
      | 'SumMode', 'KeepLSB', 'SumWordLength', 32,...
      | 'CastBeforeSum', false)
  data: Pac input; gamma input; slip input; alfa input; Fz input; F_pac output; mu input; Vcx input; C_F output; R0 input
function [F_pac,C_F] = fcn(Pac,gamma,slip,alfa,Fz,mu,Vcx,R0)
% function for computing forces Fx, Fy and self-aligning torque Mz

% Pac   -> model structure with coeff. Pacejka 96
% slip  -> slip ratio [-] (-1:1)
% alfa  -> slip angle [rad]
% gamma -> camber [rad]
% Vcx,y velocity components of tire contact point C

% Structure building: Pacejka model coefficients
Pa_FZ0_ = Pac(1);
Pa_LFZ0 = Pac(2);
Pa_LmuV = Pac(3);
Pa_LKXK = Pac(4);
Pa_LKYA = Pac(5);
Pa_LCX_ = Pac(6);
Pa_LCY_ = Pac(7);
Pa_LEX_ = Pac(8);
Pa_LEY_ = Pac(9);
Pa_LHX_ = Pac(10);
Pa_LHY_ = Pac(11);
Pa_LVX_ = Pac(12);
Pa_LVY_ = Pac(13);
Pa_LKYG = Pac(14);
Pa_LKZG = Pac(15);
Pa_LT__ = Pac(16);
Pa_MR__ = Pac(17);
Pa_LXA_ = Pac(18);
Pa_LYK_ = Pac(19);
Pa_LVYK = Pac(20);
Pa_LS__ = Pac(21);
Pa_LCZ_ = Pac(22);
Pa_LMX_ = Pac(23);
Pa_LMY_ = Pac(24);
Pa_PCX1 = Pac(25);
Pa_PDX1 = Pac(26);
Pa_PDX2 = Pac(27);
Pa_PEX1 = Pac(28);
Pa_PEX2 = Pac(29);
Pa_PEX3 = Pac(30);
Pa_PEX4 = Pac(31);
Pa_PKX1 = Pac(32);
Pa_PKX2 = Pac(33);
Pa_PKX3 = Pac(34);
Pa_PHX1 = Pac(35);
Pa_PHX2 = Pac(36);
Pa_PVX1 = Pac(37);
Pa_PVX2 = Pac(38);
Pa_RBX1 = Pac(39);
Pa_RBX2 = Pac(40);
Pa_RCX1 = Pac(41);
Pa_RHX1 = Pac(42);
Pa_RTX1 = Pac(43);
Pa_RTX2 = Pac(44);
Pa_RTX3 = Pac(45);
Pa_QSX1 = Pac(46);
Pa_QSX2 = Pac(47);
Pa_QSX3 = Pac(48);
Pa_PCY1 = Pac(49);
Pa_PDY1 = Pac(50);
Pa_PDY2 = Pac(51);
Pa_PDY3 = Pac(52);
Pa_PEY1 = Pac(53);
Pa_PEY2 = Pac(54);
Pa_PEY3 = Pac(55);
Pa_PEY4 = Pac(56);
Pa_PKY1 = Pac(57);
Pa_PKY2 = Pac(58);
Pa_PKY3 = Pac(59);
Pa_PHY1 = Pac(60);
Pa_PHY2 = Pac(61);
Pa_PHY3 = Pac(62);
Pa_PVY1 = Pac(63);
Pa_PVY2 = Pac(64);
Pa_PVY3 = Pac(65);
Pa_PVY4 = Pac(66);
Pa_RBY1 = Pac(67);
Pa_RBY2 = Pac(68);
Pa_RBY3 = Pac(69);
Pa_RCY1 = Pac(70);
Pa_RHY1 = Pac(71);
Pa_RVY1 = Pac(72);
Pa_RVY2 = Pac(73);
Pa_RVY3 = Pac(74);
Pa_RVY4 = Pac(75);
Pa_RVY5 = Pac(76);
Pa_RVY6 = Pac(77);
Pa_PTY1 = Pac(78);
Pa_PTY2 = Pac(79);
Pa_QSY1 = Pac(80);
Pa_QSY2 = Pac(81);
Pa_QBZ1 = Pac(82);
Pa_QBZ2 = Pac(83);
Pa_QBZ3 = Pac(84);
Pa_QBZ4 = Pac(85);
Pa_QBZ5 = Pac(86);
Pa_QBZ6 = Pac(87);
Pa_QBZ9 = Pac(88);
Pa_QBZZ = Pac(89);
Pa_QCZ1 = Pac(90);
Pa_QDZ1 = Pac(91);
Pa_QDZ2 = Pac(92);
Pa_QDZ3 = Pac(93);
Pa_QDZ4 = Pac(94);
Pa_QDZ6 = Pac(95);
Pa_QDZ7 = Pac(96);
Pa_QDZ8 = Pac(97);
Pa_QDZ9 = Pac(98);
Pa_QEZ1 = Pac(99);
Pa_QEZ2 = Pac(100);
Pa_QEZ3 = Pac(101);
Pa_QEZ4 = Pac(102);
Pa_QEZ5 = Pac(103);
Pa_QHZ1 = Pac(104);
Pa_QHZ2 = Pac(105);
Pa_QHZ3 = Pac(106);
Pa_QHZ4 = Pac(107);
Pa_SSZ1 = Pac(108);
Pa_SSZ2 = Pac(109);
Pa_SSZ3 = Pac(110);
Pa_SSZ4 = Pac(111);
Pa_QTZ1 = Pac(112);

% Costants
epsi = 0.01;
eps_V = 0.1;
csi_0=1;
csi_4=1;
Amu = 10;
Pa_LmuX = mu;
Pa_LmuY = mu;

%-------------------------------- Fx pure slip ---------------------------
Cx = Pa_PCX1*Pa_LCX_;
dfz = (Fz-Pa_LFZ0*Pa_FZ0_)/(Pa_LFZ0*Pa_FZ0_);
mux = Pa_LmuX * (Pa_PDX1 + Pa_PDX2 * dfz);
Dx = mux*Fz; %*csi_1, con csi_1=1
%Shx = (Pa_PHX1+Pa_PHX2*dfz)*Pa_LHX_;
Shx = 0;
Kx = slip + Shx;
Ex = (Pa_PEX1+Pa_PEX2*dfz+Pa_PEX3*dfz^2)*(1-Pa_PEX4*sign(Kx))*Pa_LEX_;
if Ex>1 Et=1; end
Kxk = Fz*(Pa_PKX1+Pa_PKX2*dfz)*exp(Pa_PKX3*dfz)*Pa_LKXK;
Bx = Kxk/(Cx*Dx+epsi);
lam_mux  = Pa_LmuX*Amu/(1+(Amu-1)*Pa_LmuX);
SVx = Fz*(Pa_PVX1+Pa_PVX2*dfz)*(abs(Vcx)/(abs(Vcx)+eps_V))*Pa_LVX_*lam_mux; %*csi_1, con csi_1=1

% logitudinal slip stiffness (Fx slope in the origin)
C_Fk = Bx*Cx*Dx;

% longitudinal force
Fx0 = Dx*sin(Cx*atan(Bx*Kx-Ex*(Bx*Kx-atan(Bx*Kx)))) + SVx;

%---------------------------- Fy pure side slip --------------------------
seg=sign(Vcx);
if seg==0 seg=1; end
alfa_star = tan(alfa)*seg;
gam_star = sin(gamma);
Shy = (Pa_PHY1+Pa_PHY2*dfz)*Pa_LHY_+Pa_PHY3*gam_star*Pa_LKYG*csi_0+csi_4-1;
alfa_y = alfa_star + Shy;
Cy = Pa_PCY1*Pa_LCY_;
muy = Pa_LmuY*(Pa_PDY1+Pa_PDY2*dfz)*(1-Pa_PDY3*gam_star^2);
Dy = muy*Fz; %*csi_2, con csi_2=1
Ey = (Pa_PEY1+Pa_PEY2*dfz)*(1-(Pa_PEY3+Pa_PEY4*gam_star)*sign(alfa_y))*Pa_LEY_;
if Ey>1 Ey=1; end
Kya0 = Pa_PKY1*Pa_LFZ0*Pa_FZ0_*sin(2*atan(Fz/(Pa_PKY2*Pa_LFZ0*Pa_FZ0_)))*Pa_LKYA;
Kya = Kya0*(1-Pa_PKY3*gam_star^2); %*csi_3, con csi_3=1
By = Kya/(Cy*Dy+epsi);
lam_muy = Pa_LmuY*Amu/(1+(Amu-1)*Pa_LmuY);
SVy = Fz*((Pa_PVY1+Pa_PVY2*dfz)*Pa_LVY_+(Pa_PVY3+Pa_PVY4*dfz)*gam_star*Pa_LKYG )*lam_muy; %*csi_2, con csi_2=1
Kyg0 = (Pa_PHY3*Kya0+Fz*(Pa_PVY3+Pa_PVY4*dfz))*Pa_LKYG;

% cornering stiffness (Fy slope in the origin)
C_Fa = By*Cy*Dy;

% lateral force
Fy0 = Dy*sin(Cy*atan(By*alfa_y-Ey*(By*alfa_y-atan(By*alfa_y)))) + SVy;

% --------------------- Fx combined slip ------------------------------
Shxa = Pa_RHX1;
%Exa = Pa_REX1+Pa_REX2*dfz; NON esiste Pa.REX1 ne' Pa.REX2
Exa = 0;
Cxa = Pa_RCX1;
Bxa = Pa_RBX1*cos(atan(Pa_RBX2*slip))*Pa_LXA_;
alfaS = alfa_star+Shxa;
Gxa0 = cos(Cxa*atan(Bxa*Shxa-Exa*(Bxa*Shxa-atan(Bxa*Shxa))));
Gxa = cos(Cxa*atan(Bxa*alfaS-Exa*(Bxa*alfaS-atan(Bxa*alfaS))))/Gxa0;
Fx = Fx0*Gxa;

% ---------------------- Fy combined slip ------------------------------
Dvyk = muy*Fz*(Pa_RVY1+Pa_RVY2*dfz+Pa_RVY3*gam_star)*cos(atan(Pa_RVY4*alfa_star));%*csi_2, con csi_2=1
Svyk = Dvyk*sin(Pa_RVY5*atan(Pa_RVY6*slip));
Shyk = Pa_RHY1; %+Pa.RHY2*dfz; NON esiste Pa.RHY2
Cyk = Pa_RCY1;
Byk = Pa_RBY1*cos(atan(Pa_RBY2*(alfa_star-Pa_RBY3)))*Pa_LYK_;
%Eyk = Pa_REY1+Pa_REY2*dfz; NON esiste Pa.REY1 ne' Pa.REY2
Eyk = 0;
ks = slip+Shyk;
Gyk0 = cos(Cyk*atan(Byk*Shyk-Eyk*(Byk*Shyk-atan(Byk*Shyk))));
Gyk = cos(Cyk*atan(Byk*ks-Eyk*(Byk*ks-atan(Byk*ks))))/Gyk0;
Fy = Fy0*Gyk+Svyk;

% --------------------- Mz pure side slip  ---------------------------
Shf = Shy+SVy/Kya;
alfa_r = alfa_star+Shf;
Br = (Pa_QBZ9/Pa_LmuY+Pa_QBZZ*By*Cy); %*csi_6, con csi_6=1
%%% Pa_QBZZ e' in realta' QBZ10 scritto cosi' x ragioni di spazio
Cr = 1; %*csi_7, con csi_7=1
Dr = Fz*R0*((Pa_QDZ6+Pa_QDZ7*dfz)+(Pa_QDZ8+Pa_QDZ9*dfz)*gam_star)*cos(alfa)*Pa_LmuY*seg; %+csi_8-1, con csi_8=1
Mzr0 = Dr*cos(Cr*atan(Br*alfa_r));
Sht = Pa_QHZ1+Pa_QHZ2*dfz+(Pa_QHZ3+Pa_QHZ4*dfz)*gam_star;
alfa_t = alfa_star+Sht;
Bt = (Pa_QBZ1+Pa_QBZ2*dfz+Pa_QBZ3*dfz^2)*(1+Pa_QBZ5*abs(gam_star)+Pa_QBZ6*gam_star^2)*Pa_LKYA/Pa_LmuY;
if Bt<0 Bt=0; end
Ct = Pa_QCZ1;
Dt0 = Fz*R0/(Pa_LFZ0*Pa_FZ0_)*(Pa_QDZ1+Pa_QDZ2*dfz)*seg;
Dt = Dt0*(1+Pa_QDZ3*abs(gam_star)+Pa_QDZ4*gam_star^2); %*csi_5, con csi_5=1
Et = (Pa_QEZ1+Pa_QEZ2*dfz+Pa_QEZ3*dfz^2)*(1+(Pa_QEZ4+Pa_QEZ5*gam_star)*2/pi*atan(Bt*Ct*alfa_t));
if Et>1 Et=1; end
t0 = Dt*cos(Ct*atan(Bt*alfa_t - Et*(Bt*alfa_t-atan(Bt*alfa_t))))*cos(alfa);
Mz0 = -t0*Fy;
Kza0 = Dt0*Kya0;
%Kzg0 = Fz*R0*(Pa_QDZ8+Pa_QDZ9*dfz)-Dt0*Kyg0;

% aligning torque
Mz = Mz0 + Mzr0;

% ------------------------ Mz Combined -----------------------------
eps_k = 0; % 
lambda_s = Pa_LS__ ;
Fz0p = Pa_LFZ0*Pa_FZ0_;
K_yap = Kya + eps_k;
alfa_req = sqrt(alfa_r^2+(Kxk/K_yap)^2*slip^2)*sign(alfa_r);
alfa_teq = sqrt(alfa_t^2+(Kxk/K_yap)^2*slip^2)*sign(alfa_t);
s = R0*(Pa_SSZ1 + Pa_SSZ2*(Fy/Fz0p) + (Pa_SSZ3+Pa_SSZ4*dfz)*gam_star)*lambda_s;
Mzr = Dr*cos(Cr*atan(Br*alfa_req));
Fyp = Fy-Svyk; 
t = Dt*cos(Ct*atan(Bt*alfa_teq - Et*(Bt*alfa_teq-atan(Bt*alfa_teq))))*cos(alfa);
Mzp = -t*Fyp;
% aligning torque
Mz = Mzp + Mzr + s*Fx;
%%%%%%%%%%%%%%%%%%%%%%%

% Check that Fz is positive
if Fz <= 0
    Fx = 0;
    Fy = 0;
    Mz = 0;
end

% Output
F_pac = [Fx; Fy; Mz];
C_F = [C_Fk; C_Fa];

== matlab function Project_model/Front axle/map slip ==
  data: u input; slip output
function slip = fcn(u)

if isnan(u) || isinf(u)
    slip = 0;
else
    slip = u;
end

== matlab function Project_model/MATLAB Function1 ==
  data: wr input; Cr_ABS output; wf input; Cr input; Cf input; Cf_ABS output; Cregen input
function [Cr_ABS, Cf_ABS] = ABS(wr, wf, Cr, Cf, Cregen)
k = 1;
Cr_ABS = tanh(k*wr)*Cr+Cregen;
Cf_ABS = tanh(k*wf)*Cf;
end

== matlab function Project_model/Power/MATLAB Function3 ==
  data: P_mechanic input; P_electric output
function P_electric = efficiency(P_mechanic)

eta_engine = 0.9;

if P_mechanic >= 0
    P_electric = P_mechanic/eta_engine;
else 
    P_electric = P_mechanic*eta_engine;
end

== matlab function Project_model/MATLAB Function2 ==
  data: u input; y output
function y = vehicle_stopped(u)

y = 0;
if abs(u)<0.1
    y = 1;
end

== matlab function Project_model/Subsystem/MATLAB Function ==
  data: u input; y output
function y = fcn(u)

y = abs(u);
g = 9.81;

if u > 0 || abs(u)>0.2*g
    y = 0;
end
